simulink model "L1_s"  (R2023a)
settings: Solver=FixedStepAuto  StartTime=0  StopTime=4e-2  FixedStep=1e-4  RelTol=1e-3
InitFcn:
  | L = 1e-3;
  | C = 1e-3;
  | R = 2;
settings Model: Creator=LabCom  LastModifiedBy=LabCom

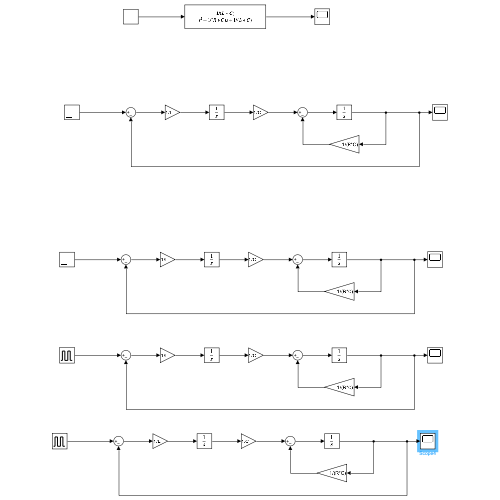
[thumbnail: Simulink's stored preview of the top-level diagram]
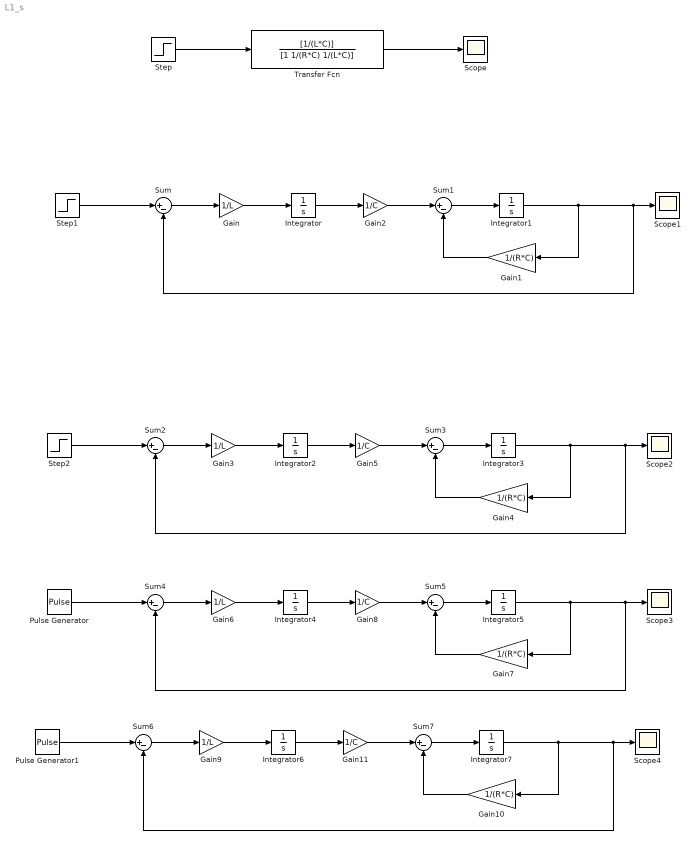
== system L1_s ==
  Gain{,3,6,9} (4 alike) : Gain  Gain=1/L
  Gain{1,4,7,10} (4 alike) : Gain  Gain=1/(R*C)
  Gain{2,5,8,11} (4 alike) : Gain  Gain=1/C
  Integrator{,1..2,4..7} (7 alike) : Integrator
  Integrator3 : Integrator  InitialCondition=1
  Pulse Generator : DiscretePulseGenerator  PulseType=Time based  Period=1/25  PulseWidth=50
  Pulse Generator1 : DiscretePulseGenerator  PulseType=Time based  Period=1/250  PulseWidth=50
  Scope{,1..4} (5 alike) : Scope
  Step : Step  Time=0  SampleTime=0
  Step1 : Step  Time=0  SampleTime=0
  Step2 : Step  Time=0  SampleTime=0
  Sum{,1..7} (8 alike) : Sum  Inputs=|+-
  Transfer Fcn : TransferFcn  Numerator=[1/(L*C)]  Denominator=[1 1/(R*C) 1/(L*C)]
  wires:
  Step/1 -> Transfer Fcn/1
  Transfer Fcn/1 -> Scope/1
  Integrator1/1 -> Sum/2, Scope1/1, Gain1/1
  Step1/1 -> Sum/1
  Sum/1 -> Gain/1
  Gain/1 -> Integrator/1
  Integrator/1 -> Gain2/1
  Gain2/1 -> Sum1/1
  Sum1/1 -> Integrator1/1
  Gain1/1 -> Sum1/2
  Gain4/1 -> Sum3/2
  Gain5/1 -> Sum3/1
  Sum3/1 -> Integrator3/1
  Integrator3/1 -> Sum2/2, Scope2/1, Gain4/1
  Integrator2/1 -> Gain5/1
  Gain3/1 -> Integrator2/1
  Step2/1 -> Sum2/1
  Sum2/1 -> Gain3/1
  Pulse Generator/1 -> Sum4/1
  Gain6/1 -> Integrator4/1
  Integrator5/1 -> Sum4/2, Scope3/1, Gain7/1
  Integrator4/1 -> Gain8/1
  Sum5/1 -> Integrator5/1
  Sum4/1 -> Gain6/1
  Gain8/1 -> Sum5/1
  Gain7/1 -> Sum5/2
  Pulse Generator1/1 -> Sum6/1
  Gain11/1 -> Sum7/1
  Gain10/1 -> Sum7/2
  Integrator6/1 -> Gain11/1
  Sum6/1 -> Gain9/1
  Gain9/1 -> Integrator6/1
  Sum7/1 -> Integrator7/1
  Integrator7/1 -> Sum6/2, Scope4/1, Gain10/1
